simulink model "disk"  (Simulink 8.7)
settings: Solver=VariableStepAuto  StartTime=0.0  StopTime=5  FixedStep=0.001  RelTol=1e-3
settings Model: Creator=Dinis  LastModifiedBy=Dinis
settings DataIOCC: LimitDataPoints=off  SaveFormat=Dataset
settings DebuggingCC: UnderspecifiedInitializationDetection=Simplified  MergeDetectMultiDrivingBlocksExec=error
settings HardwareCC: ProdBitPerPointer=64  ProdLargestAtomicFloat=Float  ProdIntDivRoundTo=Zero  ProdEndianess=LittleEndian  ProdWordSize=64  ProdHWDeviceType=Intel->x86-64 (Windows64)
settings ModelReferenceCC: PropagateSignalLabelsOutOfModel=on
settings ConfigComp: CovModelRefEnable=off

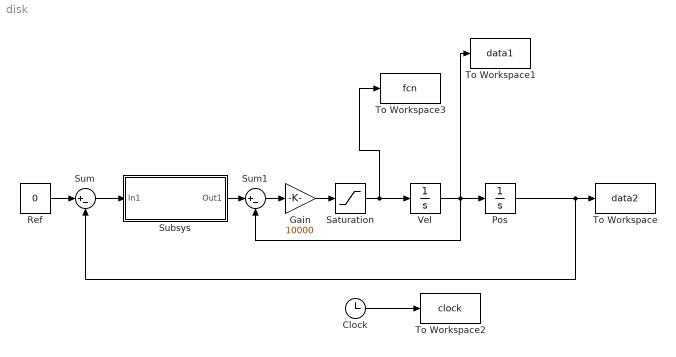
== system disk ==
  Clock : Clock
  Gain : Gain  Gain=10000
  Pos : Integrator  InitialCondition=1
  Ref : Constant  Value=0
  Saturation : Saturate  UpperLimit=1  LowerLimit=-1  ZeroCross=off
  Subsys : Subsystem
  Sum : Sum  Inputs=|+-
  Sum1 : Sum  Inputs=|+-
  To Workspace : ToWorkspace  VariableName=data2  SampleTime=-1
  To Workspace1 : ToWorkspace  VariableName=data1  SampleTime=-1
  To Workspace2 : ToWorkspace  VariableName=clock  SampleTime=-1
  To Workspace3 : ToWorkspace  VariableName=fcn  SampleTime=-1
  Vel : Integrator
  wires:
  Subsys/1(Out1) -> Sum1/1
  Sum/1 -> Subsys/1(In1)
  Ref/1 -> Sum/1
  Pos/1 -> To Workspace/1, Sum/2
  Vel/1 -> Sum1/2, To Workspace1/1, Pos/1
  Saturation/1 -> Vel/1, To Workspace3/1
  Gain/1 -> Saturation/1
  Sum1/1 -> Gain/1
  Clock/1 -> To Workspace2/1

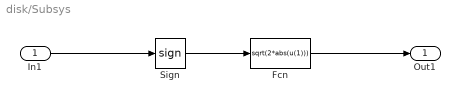
== system disk/Subsys ==
  In1 : Inport
  Fcn : Fcn  Expr=sqrt(2*abs(u(1)))
  Sign : Signum
  Out1 : Outport
  wires:
  In1/1 -> Sign/1
  Sign/1 -> Fcn/1
  Fcn/1 -> Out1/1
